simulink model "forwardfeed"  (R2019a)
settings: Solver=FixedStepAuto  StartTime=0.0  StopTime=2  FixedStep=0.1  RelTol=1e-3
values from neighbouring files (symbols this model uses):
  wn = 13.14    [meter.m]
  zeta = 0.4733    [meter.m]
undefined symbols (not defined in the file or in its folder): wn2, zeta2
settings Model: Creator=jk  LastModifiedBy=jk

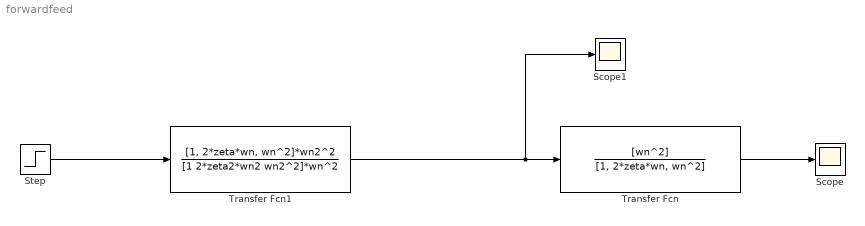
== system forwardfeed ==
  Scope : Scope
  Scope1 : Scope
  Step : Step  SampleTime=0
  Transfer Fcn : TransferFcn  Numerator=[wn^2]  Denominator=[1, 2*zeta*wn, wn^2]
  Transfer Fcn1 : TransferFcn  Numerator=[1, 2*zeta*wn, wn^2]*wn2^2  Denominator=[1 2*zeta2*wn2 wn2^2]*wn^2
  wires:
  Transfer Fcn/1 -> Scope/1
  Step/1 -> Transfer Fcn1/1
  Transfer Fcn1/1 -> Scope1/1, Transfer Fcn/1
